simulink model "ProyectoGlobal_AyCD_Cantu_LagoTejo_OPCUA"  (R2021a)
settings: Solver=ode23  StartTime=0.0  StopTime=inf  MinStep=1e-4
values from neighbouring files (symbols this model uses):
  a_hMax = 0.75    [Datos_ProyectoGlobal_AyCD_Cantu_LagoTejo.m]    (also in Datos_v18.m; PID_calculado.mat)
  a_tMax = 0.8    [Datos_ProyectoGlobal_AyCD_Cantu_LagoTejo.m]    (also in Datos_v18.m; PID_calculado.mat)
  b_cx = 1e6    (= 1000000)    [Datos_ProyectoGlobal_AyCD_Cantu_LagoTejo.m]    (also in Datos_v18.m; PID_calculado.mat)
  b_cy = 1e7    (= 10000000)    [Datos_ProyectoGlobal_AyCD_Cantu_LagoTejo.m]    (also in Datos_v18.m; PID_calculado.mat)
  b_eq_h = ((b_hd + b_hm*(i_h^2))*2/(r_hd^2))    (= 31004.4444444)    [Datos_ProyectoGlobal_AyCD_Cantu_LagoTejo.m]    (also in Datos_v18.m; PID_calculado.mat)
  b_eq_t = ((b_td + b_tm*(i_t^2))/(r_td^2))    (= 21607.2)    [Datos_ProyectoGlobal_AyCD_Cantu_LagoTejo.m]    (also in Datos_v18.m; PID_calculado.mat)
  b_hb = 1e8    (= 100000000)    [Datos_ProyectoGlobal_AyCD_Cantu_LagoTejo.m]    (also in Datos_v18.m; PID_calculado.mat)
  b_hEb = 2.2e9    (= 2200000000)    [Datos_ProyectoGlobal_AyCD_Cantu_LagoTejo.m]    (also in Datos_v18.m; PID_calculado.mat)
  b_t = 90    [Datos_ProyectoGlobal_AyCD_Cantu_LagoTejo.m]    (also in Datos_v18.m; PID_calculado.mat)
  b_tb = 5e6    (= 5000000)    [Datos_ProyectoGlobal_AyCD_Cantu_LagoTejo.m]    (also in Datos_v18.m; PID_calculado.mat)
  b_tw = 3e3    (= 3000)    [Datos_ProyectoGlobal_AyCD_Cantu_LagoTejo.m]    (also in Datos_v18.m; PID_calculado.mat)
  b_wu = 150    [Datos_ProyectoGlobal_AyCD_Cantu_LagoTejo.m]    (also in Datos_v18.m; PID_calculado.mat)
  bah = M_eq_h*n_h*omega_h    [PID_Izaje_B.m]    (also in PID_calculado.mat = 387555.555556)
  bat = M_eq_t*n_t*omega_t    [PID_Carro_B.m]    (also in PID_calculado.mat = 270090)
  CI_h = 5    [Datos_ProyectoGlobal_AyCD_Cantu_LagoTejo.m]    (also in Datos_v18.m; PID_calculado.mat)
  CI_t = -16.25    [Datos_ProyectoGlobal_AyCD_Cantu_LagoTejo.m]    (also in Datos_v18.m; PID_calculado.mat)
  g = 9.80665    [Datos_ProyectoGlobal_AyCD_Cantu_LagoTejo.m]    (also in Datos_v18.m; PID_calculado.mat)
  H_c = 2.5    [Datos_ProyectoGlobal_AyCD_Cantu_LagoTejo.m]    (also in Datos_v18.m; PID_calculado.mat)
  i_h = 22    [Datos_ProyectoGlobal_AyCD_Cantu_LagoTejo.m]    (also in Datos_v18.m; PID_calculado.mat)
  i_t = 30    [Datos_ProyectoGlobal_AyCD_Cantu_LagoTejo.m]    (also in Datos_v18.m; PID_calculado.mat)
  k_cy = 1.8e9    (= 1800000000)    [Datos_ProyectoGlobal_AyCD_Cantu_LagoTejo.m]    (also in Datos_v18.m; PID_calculado.mat)
  k_tw = 4.8e5    (= 480000)    [Datos_ProyectoGlobal_AyCD_Cantu_LagoTejo.m]    (also in Datos_v18.m; PID_calculado.mat)
  k_wu = 2.36e8    (= 236000000)    [Datos_ProyectoGlobal_AyCD_Cantu_LagoTejo.m]    (also in Datos_v18.m; PID_calculado.mat)
  Kd_bal = [-2.22044604925e-16 2.22044604925e-16 2.22044604925e-16 0 0 0 0 0 -2.22044604925e-16 0 2.22044604925e-16 -2.22044604925e-16 ... (296091 elements, 501x591)]    [Kp_Kd_balanceo.mat]    (also in PD_Balanceo.m = zeros(length(ML),length(L)))
  Kp_bal = [5.11381136401 5.1081388039 5.10248507909 5.09685008556 5.09123372013 5.08563588037 5.08005646467 5.07449537218 5.06895250283 5.06342775732 5.05792103709 5.05243224433 ... (296091 elements, 501x591)]    [Kp_Kd_balanceo.mat]    (also in PD_Balanceo.m = Kd_bal)
  ksah = M_eq_h*n_h*(omega_h^2)    [PID_Izaje_B.m]    (also in PID_calculado.mat = 922348.374575)
  ksat = M_eq_t*n_t*(omega_t^2)    [PID_Carro_B.m]    (also in PID_calculado.mat = 972648.108)
  ksiah = M_eq_h*n_h*(omega_h^3)    [PID_Izaje_B.m]    (also in PID_calculado.mat = 2195108.57705)
  ksiat = M_eq_t*n_t*(omega_t^3)    [PID_Carro_B.m]    (also in PID_calculado.mat = 3502700.36653)
  lim_xDer = 50    [Datos_ProyectoGlobal_AyCD_Cantu_LagoTejo.m]    (also in Datos_v18.m; PID_calculado.mat)
  lim_xDer_ult = 51    [Datos_ProyectoGlobal_AyCD_Cantu_LagoTejo.m]    (also in Datos_v18.m; PID_calculado.mat)
  lim_xIzq = -30    [Datos_ProyectoGlobal_AyCD_Cantu_LagoTejo.m]    (also in Datos_v18.m; PID_calculado.mat)
  lim_xIzq_ult = -31    [Datos_ProyectoGlobal_AyCD_Cantu_LagoTejo.m]    (also in Datos_v18.m; PID_calculado.mat)
  lim_yInf = -20    [Datos_ProyectoGlobal_AyCD_Cantu_LagoTejo.m]    (also in Datos_v18.m; PID_calculado.mat)
  lim_yInf_ult = -21    [Datos_ProyectoGlobal_AyCD_Cantu_LagoTejo.m]    (also in Datos_v18.m; PID_calculado.mat)
  lim_ySup = 40    [Datos_ProyectoGlobal_AyCD_Cantu_LagoTejo.m]    (also in Datos_v18.m; PID_calculado.mat)
  lim_ySup_ult = 41    [Datos_ProyectoGlobal_AyCD_Cantu_LagoTejo.m]    (also in Datos_v18.m; PID_calculado.mat)
  M_cMax = 50000    [Datos_ProyectoGlobal_AyCD_Cantu_LagoTejo.m]    (also in Datos_v18.m; PID_calculado.mat)
  M_cMin = 2000    [Datos_ProyectoGlobal_AyCD_Cantu_LagoTejo.m]    (also in Datos_v18.m; PID_calculado.mat)
  M_eq_h = (J_hd_hEb+J_hm_hb*i_h^2)*2/r_hd^2    (= 65137.7777778)    [Datos_ProyectoGlobal_AyCD_Cantu_LagoTejo.m]    (also in Datos_v18.m; PID_calculado.mat)
  M_eq_t = ((J_td + J_tm_tb*(i_t^2))/(r_td^2))    (= 30000)    [Datos_ProyectoGlobal_AyCD_Cantu_LagoTejo.m]    (also in Datos_v18.m; PID_calculado.mat)
  M_s = 15000    [Datos_ProyectoGlobal_AyCD_Cantu_LagoTejo.m]    (also in Datos_v18.m; PID_calculado.mat)
  M_t = 30000    [Datos_ProyectoGlobal_AyCD_Cantu_LagoTejo.m]    (also in Datos_v18.m; PID_calculado.mat)
  r_hd = 0.75    [Datos_ProyectoGlobal_AyCD_Cantu_LagoTejo.m]    (also in Datos_v18.m; PID_calculado.mat)
  r_td = 0.5    [Datos_ProyectoGlobal_AyCD_Cantu_LagoTejo.m]    (also in Datos_v18.m; PID_calculado.mat)
  T_hbMax = 5e4    (= 50000)    [Datos_ProyectoGlobal_AyCD_Cantu_LagoTejo.m]    (also in Datos_v18.m; PID_calculado.mat)
  T_hEbMax = 1.1e6    (= 1100000)    [Datos_ProyectoGlobal_AyCD_Cantu_LagoTejo.m]    (also in Datos_v18.m; PID_calculado.mat)
  T_hmMax = 2e4    (= 20000)    [Datos_ProyectoGlobal_AyCD_Cantu_LagoTejo.m]    (also in Datos_v18.m; PID_calculado.mat)
  T_tbMax = 5e3    (= 5000)    [Datos_ProyectoGlobal_AyCD_Cantu_LagoTejo.m]    (also in Datos_v18.m; PID_calculado.mat)
  T_tmMax = 3e3    (= 3000)    [Datos_ProyectoGlobal_AyCD_Cantu_LagoTejo.m]    (also in Datos_v18.m; PID_calculado.mat)
  tau_hm = 1e-3    (= 0.001)    [Datos_ProyectoGlobal_AyCD_Cantu_LagoTejo.m]    (also in Datos_v18.m; PID_calculado.mat)
  tau_tm = 1e-3    (= 0.001)    [Datos_ProyectoGlobal_AyCD_Cantu_LagoTejo.m]    (also in Datos_v18.m; PID_calculado.mat)
  v_hMax_0 = 3    [Datos_ProyectoGlobal_AyCD_Cantu_LagoTejo.m]    (also in Datos_v18.m; PID_calculado.mat)
  v_tMax = 4    [Datos_ProyectoGlobal_AyCD_Cantu_LagoTejo.m]    (also in Datos_v18.m; PID_calculado.mat)
  xc = [-28.75 -26.25 -23.75 -21.25 -18.75 -16.25 -13.75 -11.25 -8.75 -6.25 -3.75 -1.25 ... (32 elements, 1x32)]    [PID_calculado.mat]    (also in Perfil_Carga.m = -30+1.25:2.5:50-1.25)
  Y_t0 = 45    [Datos_ProyectoGlobal_AyCD_Cantu_LagoTejo.m]    (also in Datos_v18.m; PID_calculado.mat)
  yc = [0 0 0 2.5 0 2.5 0 2.5 0 0 0 0 ... (32 elements, 1x32)]    [PID_calculado.mat]    (also in Perfil_Carga.m = yc2)
undefined symbols (not defined in the file or in its folder): bcx, bcy, Cond_Ini_h, Cond_Ini_t, Kcy
libraries: simulink x13, opclib x3
(part 3 of 3)

== matlab function ProyectoGlobal_AyCD_Cantu_LagoTejo_OPCUA/Modelo Fisico Carro-Izaje-Carga/Modos de Contacto/MATLAB Function2 ==
  data: Susp input; Y_c0 output; x_l input; yc_act output; yc input; TLK input; TLK_ant input; change output; yc_act_ant input
function [Y_c0,yc_act,change] = update_yc(Susp,x_l,yc,TLK,TLK_ant,yc_act_ant)
%Susp -> modo de contacto (1 suspendido , 0 apoyado)
change=0;

%Posicionamiento de container en el plano
idx=1;
for i=1:length(yc(1,:))
    if ((x_l>=(yc(1,i)-1.25))&&(x_l<(yc(1,i)+1.25)))
        idx = i;
    end
end


if(yc_act_ant == yc)
    %Cierra el Twistlock -> Container tomado(Se quita del suelo)
    if((TLK==1) && (TLK_ant==0) && (Susp==0))

        if(x_l>2.5 && x_l <47.5)   

            if(yc(2,idx)>-20 )
                yc(2,idx) = yc(2,idx) - 2.5;
            end
            yc_act = yc;
            Y_c0 = yc_act(2,idx);
            change=1;

        elseif(x_l>-37.5 && x_l <-2.5)

            if(yc(2,idx)>0 )
                yc(2,idx) = yc(2,idx) - 2.5;
            end
            yc_act = yc;
            Y_c0 = yc_act(2,idx);
            change=1;

        end

    %Abre el Twistlock -> Container posicionado y soltado(Se agrega al suelo)
    elseif((TLK==0) && (TLK_ant==1) && (Susp==0))
        if(yc(2,idx)<32.5 )
            yc(2,idx) = yc(2,idx) + 2.5;        
        end
        yc_act = yc;
        Y_c0 = yc_act(2,idx);
        change=1;
    else
        change=0;
    end
    
end

yc_act = yc;
Y_c0 = yc_act(2,idx);

end

== matlab function ProyectoGlobal_AyCD_Cantu_LagoTejo_OPCUA/Modelo Fisico Carro-Izaje-Carga/Modos de Contacto/MATLAB Function1 ==
  data: Susp input; Y_c0 output size=1; x_l input; Yc input; Xc input; TLK input; TLKold input; yc_act_old input size=[1 32]; yc_act output size=[1 32]; change output size=1
function [Y_c0,yc_act,  change] = yc_actual(Susp,x_l,Yc,Xc,TLK,TLKold,yc_act_old)
%Susp: modo de contacto (1 suspendido , 0 apoyado)
change=0;

%yc_act = zeros(1,length(yc));
%Posicionamiento de container en el plano
idx=1;

for i=1:length(Xc)
    if ((x_l>=(Xc(i)-1.25))&&(x_l<(Xc(i)+1.25)))
        idx = i;
    end
end

if(yc_act_old == Yc)
    %Cierra el Twistlock -> Container tomado(Se quita del suelo)
    if((TLK==1) && (TLKold==0) && (Susp==0))
        
        if(x_l>2.5 && x_l<47.5)
            
            if(Yc(idx)>-20 )
                Yc(idx) = Yc(idx) - 2.5;
            end
            yc_act = Yc;
            Y_c0 = yc_act(idx);
            change=1;
            
        elseif(x_l>-37.5 && x_l <-2.5)
            
            if(Yc(idx)>0)
                Yc(idx) = Yc(idx) - 2.5;
            end
            yc_act = Yc;
            Y_c0 = yc_act(idx);
            change=1;
            
        end
        
        %Abre el Twistlock -> Container posicionado y soltado(Se agrega al suelo)
    elseif((TLK==0) && (TLKold==1) && (Susp==0))
        if(Yc(idx)<32.5 )
            Yc(idx) = Yc(idx) + 2.5;
        end
        yc_act = Yc;
        Y_c0 = yc_act(idx);
        change=1;
    else
        change=0;
    end
    
end




yc_act = Yc;
Y_c0 = yc_act(idx);
end

== matlab function ProyectoGlobal_AyCD_Cantu_LagoTejo_OPCUA/Nivel 2/MATLAB Function ==
  data: m_l input; l_h input; Kp output; Kd output; kd_bal input; kp_bal input
function [Kp,Kd] = fcn(m_l,l_h,kd_bal,kp_bal)
index_ml = ceil(m_l/100);
index_h = ceil(l_h/0.1);
if(index_ml <= 1)
   index_ml = 1; 
end

if(index_h <= 1)
   index_h = 1; 
end

if(index_ml >= 51)
   index_ml = 51; 
end

if(index_h >= 60)
   index_h = 60; 
end
Kd = kd_bal(index_ml,index_h);
Kp = kp_bal(index_ml,index_h);

end
